simulink model "lqr_controller"  (R2024b)
settings: Solver=ode4  StartTime=0.0  StopTime=12  FixedStep=0.001  RelTol=1e-3
values from neighbouring files (symbols this model uses):
  K_matrix = [K_matrix; K]    [getting_lqr_gain.m]
  v_initial = v(1)    [analytic_simulation.m]    (also in lqr_simulation.m = 15; ref_traj_generator.m = 15)
  V_vect = (5:1:30)'    [getting_lqr_gain.m]
undefined symbols (not defined in the file or in its folder): path
libraries: autolibutils x4, autolibshared x2, vehdynlibsteering x1, simulink x1, SignalEditorBlockLib x1
(part 1 of 3)
settings Model: Creator=jeongheon  LastModifiedBy=junhyeongdoh
settings RTWCC: GPUComputeCapability=3.5

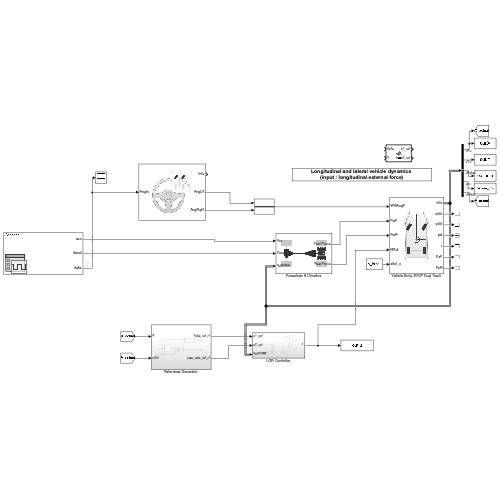
[thumbnail: Simulink's stored preview of the top-level diagram]
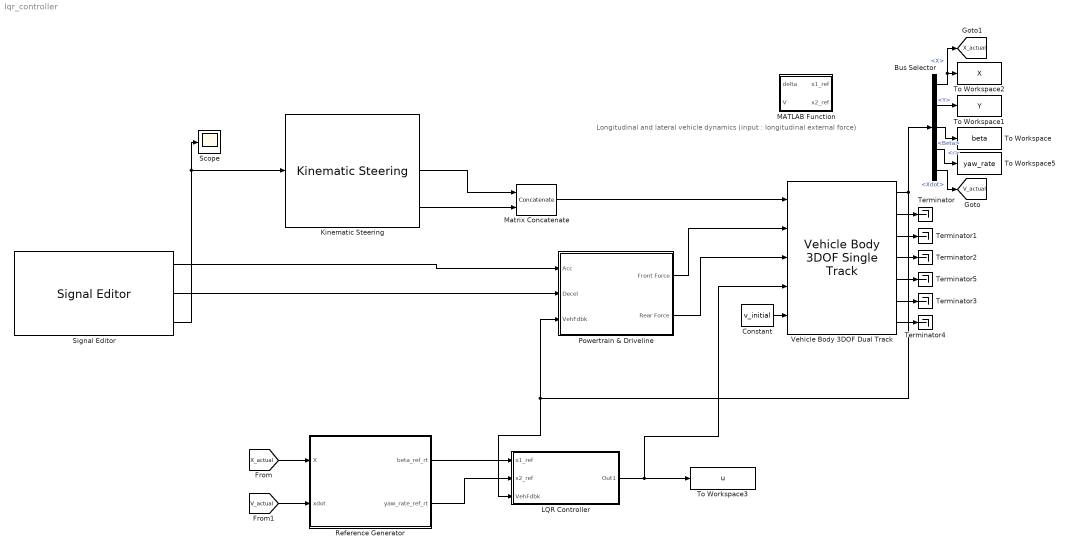
== system lqr_controller ==
  note: Longitudinal and lateral vehicle dynamics
      | (input : longitudinal external force)
  Bus Selector : BusSelector  OutputSignals=InertFrm.Cg.Disp.X,InertFrm.Cg.Disp.Y,BdyFrm.Cg.Ang.Beta,BdyFrm.Cg.AngVel.r,InertFrm.Cg.Vel.Xdot
  Constant : Constant  Value=v_initial
  Kinematic Steering : vehdynlibsteering/Kinematic Steering  StrgType=Ackerman  StrgRatioType=Constant  Loc=Front  NrmlFctr=0.01  TrckWdth=1.4  WhlBase=3  Db=0  StrgRng=1.25*pi  StrgAngBpts="[-6.2832   -5.0265   -3.7699   -2.5133   -1.2566         0    1.2566    2.5133    3.7699    5.0265    6.2832]"  StrgRatioTbl=|  StrgRatio=1  PctAckIn=off  PctAck=100  PctAckTbl=ones(1,11)*100  StrgArmLngth=0.1  RckCsLngth=0.5  TieRodLngth=0.248  D=0.2  PnnRadius=0.00085818  PnnRadiusTbl="[0.0055    0.0055    0.0056    0.0057    0.0058    0.0057    0.0057    0.0057    0.0056    0.0055    0.0055]"  RodLngth=0.1  ParaArmLngth=0.9  aMode=2
      | [13.5000   13.3750   13.2500   13.1250   13.0000   13.0000   13.0000   13.1250   13.2500   13.3750   13.5000
      | ]
  LQR Controller : Subsystem
  MATLAB Function : MATLAB Function  TreatAsAtomicUnit=on
  Matrix Concatenate : Concatenate  ConcatenateDimension=2
  Powertrain & Driveline : Subsystem
      mask Display: image('vdbslibpt.png');
  Reference Generator : Subsystem
  Scope : Scope
  Signal Editor : SignalEditorBlockLib/Signal Editor  FileName=accdelta.mat  ActiveScenario=Scenario  ActiveSignal=acc  IsBus=off  OutputBusObjectStr=Bus: BusObject  SampleTime=0  Interpolate=off  ZeroCross=off  OutputAfterFinalValue=Setting to zero  Unit=inherit  PreserveSignalName=on  ApplySigPropsToAllScenarios=off  ApplySigPropsToAllSignals=off
  Terminator{,1..5} (6 alike) : Terminator
  To Workspace : ToWorkspace  VariableName=beta  SaveFormat=Timeseries  SampleTime=-1
  To Workspace1 : ToWorkspace  VariableName=Y  SaveFormat=Timeseries  SampleTime=-1
  To Workspace2 : ToWorkspace  VariableName=X  SaveFormat=Timeseries  SampleTime=-1
  To Workspace3 : ToWorkspace  VariableName=u  SaveFormat=Timeseries  SampleTime=-1
  To Workspace5 : ToWorkspace  VariableName=yaw_rate  SaveFormat=Timeseries  SampleTime=-1
  Vehicle Body 3DOF Dual Track : autolibshared/Vehicle Body 3DOF Single Track  trackMode=Dual  inputMode=External longitudinal forces  frontSteerMode=on  rearSteerMode=off  windMode=off  muMode=off  extFMode=off  extMMode=on  htchFMode=off  htchMMode=off  extXo=off  extpsio=off  extxdoto=on  extro=off  extYo=off  extTamb=off  extydoto=off  aMode=2  NF=2  NR=2  m=2000  a=1.4  b=1.6  h=0.35  dh=1  hh=0.2  X_o=0  xdot_o=15  CalphaMode=off  sigmaMode=on  d=0  hl=0  w=[1.4,1.4]  Cy_f=12e3  Cy_r=11e3  sigma_f=.1  sigma_r=.1  alpha_f_brk=[-.1 .1]  Cy_f_data=[-9e3 9e3]  alpha_r_brk=[-.1 .1]  Cy_r_data=[-9e3 9e3]  Y_o=0  ydot_o=0  Izz=4000  psi_o=0  r_o=0  Af=2  Cd=.3  Cl=.1  Cpm=.1  beta_w=[0:0.01:0.3]  Cs=[0:0.03:0.9]  Cym=[0:0.01:0.3]  Pabs=101325  Tair=273  g=9.81  mu=1  xdot_tol=.01  Fznom=5000  Fxtire_sat=7e4  Fytire_sat=7e4  longOff=0  latOff=0  vertOff=0  wrapAng=off
  tag scope: V_actual=global, X_actual=global
  wires:
  Kinematic Steering/3 -> Matrix Concatenate/2
  Kinematic Steering/2 -> Matrix Concatenate/1
  Signal Editor/1 -> Powertrain & Driveline/1(Acc)
  Vehicle Body 3DOF Dual Track/2 -> Terminator/1
  Matrix Concatenate/1 -> Vehicle Body 3DOF Dual Track/1
  Vehicle Body 3DOF Dual Track/4 -> Terminator2/1
  Vehicle Body 3DOF Dual Track/7 -> Terminator4/1
  Vehicle Body 3DOF Dual Track/6 -> Terminator3/1
  Vehicle Body 3DOF Dual Track/3 -> Terminator1/1
  Powertrain & Driveline/2(Rear Force) -> Vehicle Body 3DOF Dual Track/3
  Powertrain & Driveline/1(Front Force) -> Vehicle Body 3DOF Dual Track/2
  Vehicle Body 3DOF Dual Track/5 -> Terminator5/1
  Vehicle Body 3DOF Dual Track/1 -> Powertrain & Driveline/3(VehFdbk), LQR Controller/3(VehFdbk), Bus Selector/1
  Signal Editor/2 -> Powertrain & Driveline/2(Decel)
  Bus Selector/1 -> [X_actual], To Workspace2/1  "<X>"
  Bus Selector/2 -> To Workspace1/1  "<Y>"
  Bus Selector/3 -> To Workspace/1  "<Beta>"
  Bus Selector/4 -> To Workspace5/1  "<r>"
  Constant/1 -> Vehicle Body 3DOF Dual Track/5
  Signal Editor/3 -> Scope/1, Kinematic Steering/1
  LQR Controller/1(Out1) -> Vehicle Body 3DOF Dual Track/4, To Workspace3/1
  Bus Selector/5 -> [V_actual]  "<Xdot>"
  [X_actual] -> Reference Generator/1(X)
  [V_actual] -> Reference Generator/2(xdot)
  Reference Generator/1(beta_ref_rt) -> LQR Controller/1(x1_ref)
  Reference Generator/2(yaw_rate_ref_rt) -> LQR Controller/2(x2_ref)

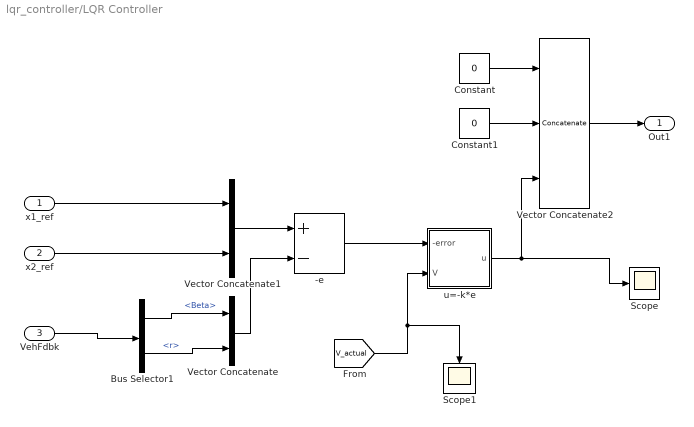
== system lqr_controller/LQR Controller ==
  x1_ref : Inport
  x2_ref : Inport  Port=2
  VehFdbk : Inport  Port=3
  -e : Sum  Inputs=+-
  Bus Selector1 : BusSelector  OutputSignals=BdyFrm.Cg.Ang.Beta,BdyFrm.Cg.AngVel.r
  Constant : Constant  Value=0
  Constant1 : Constant  Value=0
  Scope : Scope
  Scope1 : Scope
  Vector Concatenate : Concatenate
  Vector Concatenate1 : Concatenate
  Vector Concatenate2 : Concatenate  NumInputs=3
  u=-k*e : Subsystem
  Out1 : Outport
  wires:
  x2_ref/1 -> Vector Concatenate1/2
  Bus Selector1/1 -> Vector Concatenate/1  "<Beta>"
  VehFdbk/1 -> Bus Selector1/1
  [V_actual] -> Scope1/1, u=-k*e/2(V)
  Vector Concatenate/1 -> -e/2
  Bus Selector1/2 -> Vector Concatenate/2  "<r>"
  -e/1 -> u=-k*e/1(-error)
  Vector Concatenate1/1 -> -e/1
  Constant/1 -> Vector Concatenate2/1
  Constant1/1 -> Vector Concatenate2/2
  u=-k*e/1("u ") -> Vector Concatenate2/3, Scope/1
  x1_ref/1 -> Vector Concatenate1/1
  Vector Concatenate2/1 -> Out1/1

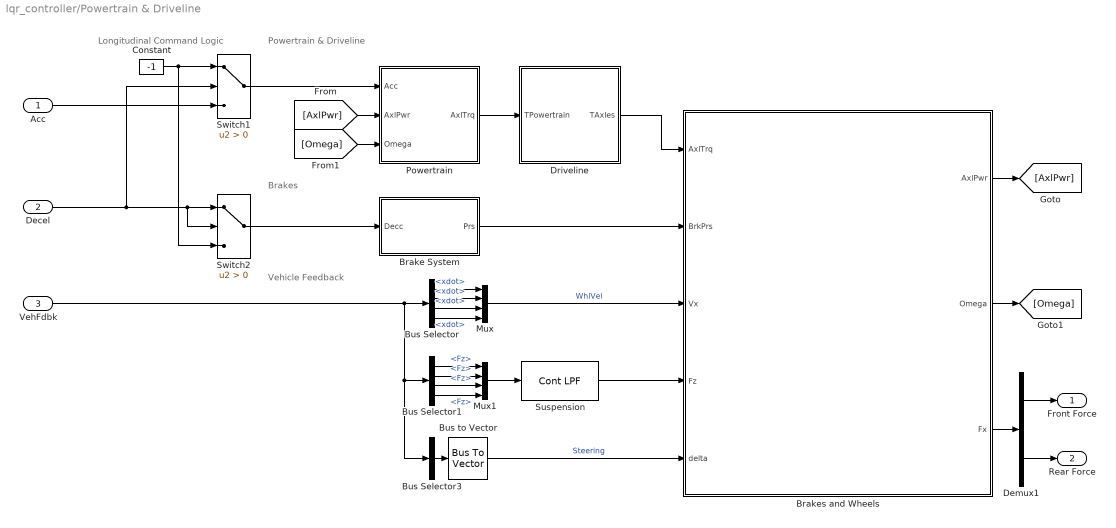
== system lqr_controller/Powertrain & Driveline ==
  note: Vehicle Feedback
  note: Powertrain & Driveline
  note: Brakes
  note: Longitudinal Command Logic
  Acc : Inport
  Decel : Inport  Port=2
  VehFdbk : Inport  Port=3
  Brake System : Subsystem
  Brakes and Wheels : Subsystem  TreatAsAtomicUnit=on
      mask Display: image('vdbslibwhls.png');
  Bus Selector : BusSelector  OutputSignals=BdyFrm.FrntAxl.Lft.Vel.xdot,BdyFrm.FrntAxl.Rght.Vel.xdot,BdyFrm.RearAxl.Lft.Vel.xdot,BdyFrm.RearAxl.Rght.Vel.xdot
  Bus Selector1 : BusSelector  OutputSignals=BdyFrm.Forces.FrntAxl.Lft.Fz,BdyFrm.Forces.FrntAxl.Rght.Fz,BdyFrm.Forces.RearAxl.Lft.Fz,BdyFrm.Forces.RearAxl.Rght.Fz
  Bus Selector3 : BusSelector  OutputSignals=BdyFrm.FrntAxl.Steer.WhlAngFL,BdyFrm.FrntAxl.Steer.WhlAngFR,BdyFrm.RearAxl.Steer.WhlAngRL,BdyFrm.RearAxl.Steer.WhlAngRR  OutputAsBus=on
  Bus to Vector : BusToVector
  Constant : Constant  Value=-1
  Demux1 : Demux  Outputs=[2 2]
  Driveline : Subsystem  Variant=on  VariantControlMode=label  VariantControl=Variant1  LabelModeActiveChoice=0
  Mux : Mux
  Mux1 : Mux
  Powertrain : Subsystem
  Suspension : autolibutils/Cont LPF  wc=10*pi*2  AbsoluteTolerance=auto  aMode=2
  Switch1 : Switch  Criteria=u2 > Threshold  SaturateOnIntegerOverflow=off  InputSameDT=off
  Switch2 : Switch  Criteria=u2 > Threshold  SaturateOnIntegerOverflow=off  InputSameDT=off
  Front Force : Outport  VectorParamsAs1DForOutWhenUnconnected=off
  Rear Force : Outport  Port=2  VectorParamsAs1DForOutWhenUnconnected=off
  wires:
  Brake System/1(Prs) -> Brakes and Wheels/2(BrkPrs)
  Switch2/1 -> Brake System/1(Decc)
  [Omega] -> Powertrain/3(Omega)
  [AxlPwr] -> Powertrain/2(AxlPwr)
  Brakes and Wheels/2(Omega) -> [Omega]
  Powertrain/1(AxlTrq) -> Driveline/1(TPowertrain)
  Switch1/1 -> Powertrain/1(Acc)
  Bus Selector1/4 -> Mux1/4  "<Fz>"
  Bus Selector1/3 -> Mux1/3  "<Fz>"
  Bus Selector1/2 -> Mux1/2  "<Fz>"
  Bus Selector1/1 -> Mux1/1  "<Fz>"
  Bus Selector/4 -> Mux/4  "<xdot>"
  Bus Selector/3 -> Mux/3  "<xdot>"
  Bus Selector/2 -> Mux/2  "<xdot>"
  Bus Selector/1 -> Mux/1  "<xdot>"
  Suspension/1 -> Brakes and Wheels/4(Fz)
  Mux1/1 -> Suspension/1
  Bus to Vector/1 -> Brakes and Wheels/5(delta)  "Steering"
  Bus Selector3/1 -> Bus to Vector/1
  Brakes and Wheels/3(Fx) -> Demux1/1
  Brakes and Wheels/1(AxlPwr) -> [AxlPwr]
  Driveline/1(TAxles) -> Brakes and Wheels/1(AxlTrq)
  Demux1/2 -> Rear Force/1
  Demux1/1 -> Front Force/1
  VehFdbk/1 -> Bus Selector/1, Bus Selector1/1, Bus Selector3/1
  Mux/1 -> Brakes and Wheels/3(Vx)  "WhlVel"
  Constant/1 -> Switch1/1, Switch2/3
  Acc/1 -> Switch1/3
  Decel/1 -> Switch2/1, Switch2/2, Switch1/2

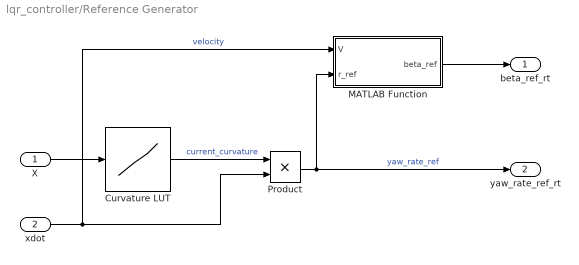
== system lqr_controller/Reference Generator ==
  X : Inport
  xdot : Inport  Port=2
  Curvature LUT : Lookup_n-D  NumberOfTableDimensions=1  BreakpointsForDimension1=path.x  Table=path.curvature  InternalRulePriority=Speed  RndMeth=Simplest
  MATLAB Function : MATLAB Function  TreatAsAtomicUnit=on
  Product : Product
  beta_ref_rt : Outport
  yaw_rate_ref_rt : Outport  Port=2
  wires:
  X/1 -> Curvature LUT/1
  Curvature LUT/1 -> Product/1  "current_curvature"
  xdot/1 -> Product/2, MATLAB Function/1(V)  "velocity"
  Product/1 -> MATLAB Function/2(r_ref), yaw_rate_ref_rt/1  "yaw_rate_ref"
  MATLAB Function/1(beta_ref) -> beta_ref_rt/1

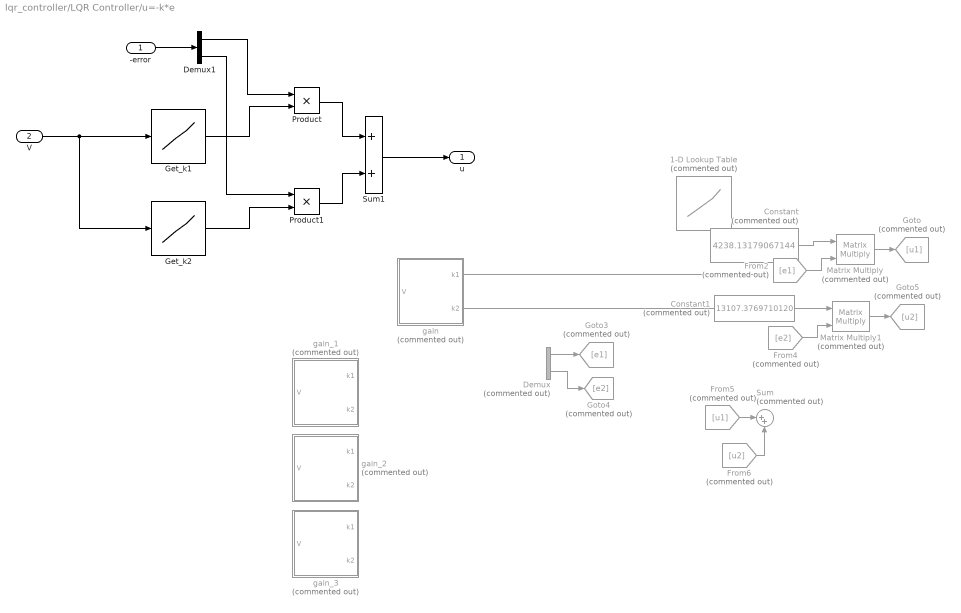
== system lqr_controller/LQR Controller/u=-k*e ==
  -error : Inport
  V : Inport  Port=2
  1-D Lookup Table : Lookup_n-D  Commented=on  NumberOfTableDimensions=1  BreakpointsForDimension1=[-5:5]  Table=tanh([-5:5])  InternalRulePriority=Speed  RndMeth=Simplest
  Constant : Constant  Commented=on  Value=4238.13179067144
  Constant1 : Constant  Commented=on  Value=13107.3769710120
  Demux : Demux  Commented=on  Outputs=2
  Demux1 : Demux  Outputs=2
  From2 : From  Commented=on  GotoTag=e1
  From4 : From  Commented=on  GotoTag=e2
  From5 : From  Commented=on  GotoTag=u1
  From6 : From  Commented=on  GotoTag=u2
  Get_k1 : Lookup_n-D  NumberOfTableDimensions=1  BreakpointsForDimension1=V_vect  Table=K_matrix(:,1)  InternalRulePriority=Speed  RndMeth=Simplest
  Get_k2 : Lookup_n-D  NumberOfTableDimensions=1  BreakpointsForDimension1=V_vect  Table=K_matrix(:,2)  InternalRulePriority=Speed  RndMeth=Simplest
  Goto : Goto  Commented=on  GotoTag=u1
  Goto3 : Goto  Commented=on  GotoTag=e1
  Goto4 : Goto  Commented=on  GotoTag=e2
  Goto5 : Goto  Commented=on  GotoTag=u2
  Matrix Multiply : Product  Commented=on  Multiplication=Matrix(*)
  Matrix Multiply1 : Product  Commented=on  Multiplication=Matrix(*)
  Product : Product
  Product1 : Product
  Sum : Sum  Commented=on  Inputs=|++
  Sum1 : Sum
  gain : MATLAB Function  Commented=on  TreatAsAtomicUnit=on
  gain_1 : MATLAB Function  Commented=on  TreatAsAtomicUnit=on
  gain_2 : MATLAB Function  Commented=on  TreatAsAtomicUnit=on
  gain_3 : MATLAB Function  Commented=on  TreatAsAtomicUnit=on
  "u " : Outport
  wires:
  Demux/1 -> Goto3/1
  Demux/2 -> Goto4/1
  gain/1(k1) -> ?
  From2/1 -> Matrix Multiply/2
  Matrix Multiply/1 -> Goto/1
  From4/1 -> Matrix Multiply1/2
  Matrix Multiply1/1 -> Goto5/1
  From6/1 -> Sum/2
  From5/1 -> Sum/1
  gain/2(k2) -> ?
  Constant/1 -> Matrix Multiply/1
  Constant1/1 -> Matrix Multiply1/1
  V/1 -> Get_k2/1, Get_k1/1
  -error/1 -> Demux1/1
  Demux1/1 -> Product/1
  Get_k1/1 -> Product/2
  Demux1/2 -> Product1/1
  Get_k2/1 -> Product1/2
  Product/1 -> Sum1/1
  Product1/1 -> Sum1/2
  Sum1/1 -> "u "/1

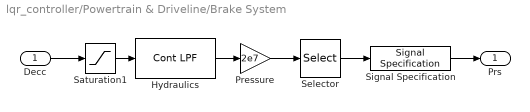
== system lqr_controller/Powertrain & Driveline/Brake System ==
  Decc : Inport
  Hydraulics : autolibutils/Cont LPF  wc=30*pi*2  AbsoluteTolerance=auto  aMode=2
  Pressure : Gain  Gain=2e7
  Saturation1 : Saturate  UpperLimit=inf  LowerLimit=0  ZeroCross=off
  Selector : Selector  InputPortWidth=1  IndexOptions=Index vector (dialog)  Indices=[1 1 1 1]  OutputSizes=1
  Signal Specification : SignalSpecification  Unit=Pa
  Prs : Outport  VectorParamsAs1DForOutWhenUnconnected=off
  wires:
  Signal Specification/1 -> Prs/1
  Decc/1 -> Saturation1/1
  Selector/1 -> Signal Specification/1
  Saturation1/1 -> Hydraulics/1
  Hydraulics/1 -> Pressure/1
  Pressure/1 -> Selector/1
